simulink model "SW_chart"  (R2023b)
settings: Solver=VariableStepAuto  StartTime=0.0  StopTime=10.0  RelTol=1e-3
settings Model: Creator=Amin  LastModifiedBy=Amin

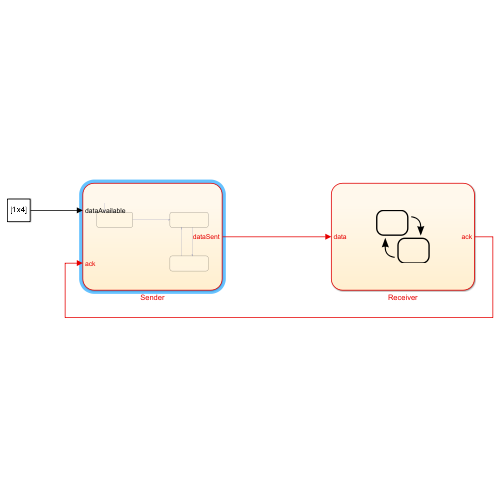
[thumbnail: Simulink's stored preview of the top-level diagram]
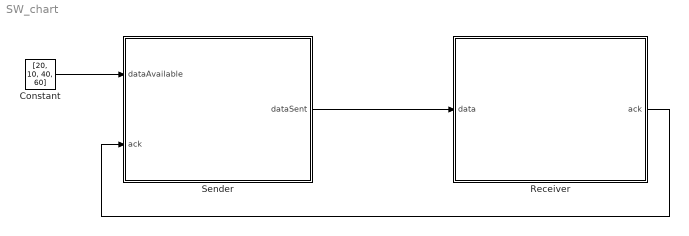
== system SW_chart ==
  Constant : Constant  Value=[20, 10, 40, 60]
  Receiver : Stateflow chart  TreatAsAtomicUnit=on
  Sender : Stateflow chart  TreatAsAtomicUnit=on
  wires:
  Constant/1 -> Sender/1(dataAvailable)
  Receiver/1(ack) -> Sender/2(ack)
  Sender/1(dataSent) -> Receiver/1(data)

== stateflow chart SW_chart/Receiver ==
  data: ack output; data input

== stateflow chart SW_chart/Sender ==
  state Idle
    dataSent = NaN
  state Send
    dataSent = dataAvailable(index)
    data = dataSent
  state WaitForAck
    dataSent = NaN
  (default) -> Idle : {data=NaN
      | index=0}
  Idle -> Send : [dataSent==data]
  WaitForAck -> Send : [ack==NaN && after(5, sec)]
  Send -> WaitForAck
  data: dataAvailable input; ack input; dataSent output; data local; index local
